simulink model "flexible_launcher_syn"  (R2020b)
settings: Solver=ode23s  StartTime=0.0  StopTime=100  FixedStep=0.05  RelTol=1e-3  EnableMultiTasking=on
undefined symbols (not defined in the file or in its folder): As, Bs, Cs, dhdx, Ds
settings Model: ExtModeAutoUpdateStatusClock=off  Creator=chiappa  LastModifiedBy=X000274
settings DataIOCC: LimitDataPoints=on  SaveFormat=Array  SignalLoggingSaveFormat=ModelDataLogs  ReturnWorkspaceOutputs=off  SignalLoggingName=sigsOut
settings OptimizationCC: BlockReduction=off  BooleanDataType=off
settings DebuggingCC: SaveWithParameterizedLinksMsg=none  UnderspecifiedInitializationDetection=Classic  MergeDetectMultiDrivingBlocksExec=none  SignalResolutionControl=TryResolveAllWithWarning  MultiTaskDSMMsg=warning  MultiTaskCondExecSysMsg=none
settings HardwareCC: ProdBitPerPointer=32  ProdBitPerSizeT=32  ProdBitPerPtrDiffT=32  ProdLargestAtomicFloat=None  ProdIntDivRoundTo=Undefined  ProdEndianess=Unspecified  ProdWordSize=32  ProdHWDeviceType=32-bit Generic  TargetUnknown=on
settings ModelReferenceCC: PropagateSignalLabelsOutOfModel=off
settings GRTTargetCC: CombineOutputUpdateFcns=off  GRTInterface=on
settings ConfigComp: CovMetricSettings=dw  CovSaveCumulativeToWorkspaceVar=on  CovSaveSingleToWorkspaceVar=on

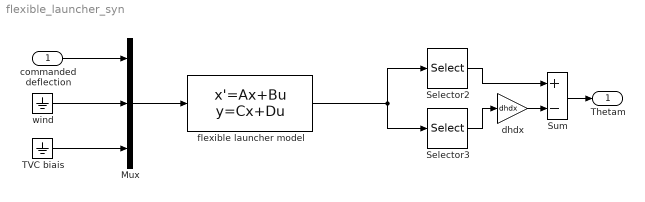
== system flexible_launcher_syn ==
  commanded deflection : Inport
  Mux : Mux  Inputs=3
  Selector2 : Selector  InputPortWidth=8  IndexOptions=Index vector (dialog)  Indices=[2]  OutputSizes=1
  Selector3 : Selector  InputPortWidth=8  IndexOptions=Index vector (dialog)  Indices=[7]  OutputSizes=1
  Sum : Sum  Inputs=+-  SaturateOnIntegerOverflow=on
  TVC biais : Ground
  dhdx : Gain  Gain=dhdx  SaturateOnIntegerOverflow=on  OutDataTypeStr=Inherit: Same as input  ParamDataTypeStr=Inherit: Same as input
  flexible launcher model : StateSpace  A=As  B=Bs  C=Cs  D=Ds  InitialCondition=0
  wind : Ground
  Thetam : Outport
  wires:
  Mux/1 -> flexible launcher model/1
  flexible launcher model/1 -> Selector2/1, Selector3/1
  commanded deflection/1 -> Mux/1
  Selector2/1 -> Sum/1
  Selector3/1 -> dhdx/1
  Sum/1 -> Thetam/1
  dhdx/1 -> Sum/2
  wind/1 -> Mux/2
  TVC biais/1 -> Mux/3
